simulink model "model_1_2_tasks"  (R2021b)
settings: Solver=FixedStepAuto  StartTime=0.0  StopTime=15  FixedStep=0.001  RelTol=1e-3
undefined symbols (not defined in the file): A1, A2, B1, B2, C1, C2, D1, D2, K1, K2, L1, L2
settings Model: Creator=den  LastModifiedBy=den

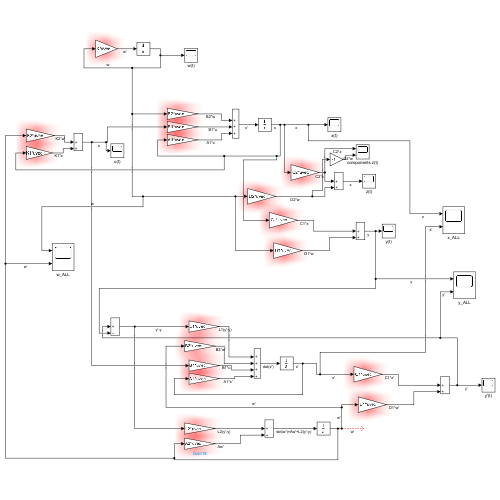
[thumbnail: Simulink's stored preview of the top-level diagram]
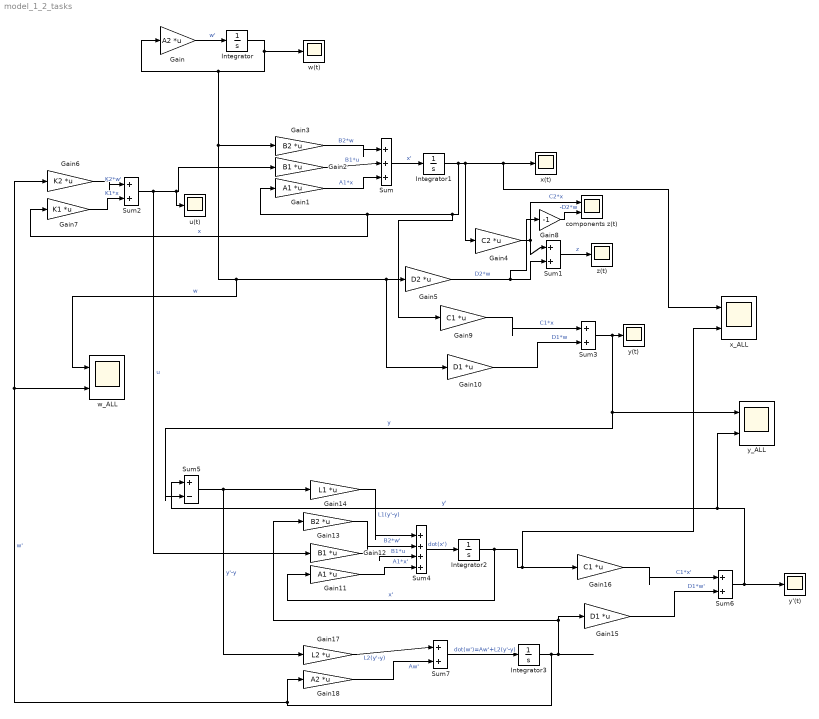
== system model_1_2_tasks ==
  Gain : Gain  Gain=A2  Multiplication=Matrix(K*u) (u vector)
  Gain1 : Gain  Gain=A1  Multiplication=Matrix(K*u) (u vector)
  Gain10 : Gain  Gain=D1  Multiplication=Matrix(K*u) (u vector)
  Gain11 : Gain  Gain=A1  Multiplication=Matrix(K*u) (u vector)
  Gain12 : Gain  Gain=B1  Multiplication=Matrix(K*u) (u vector)
  Gain13 : Gain  Gain=B2  Multiplication=Matrix(K*u) (u vector)
  Gain14 : Gain  Gain=L1  Multiplication=Matrix(K*u) (u vector)
  Gain15 : Gain  Gain=D1  Multiplication=Matrix(K*u) (u vector)
  Gain16 : Gain  Gain=C1  Multiplication=Matrix(K*u) (u vector)
  Gain17 : Gain  Gain=L2  Multiplication=Matrix(K*u) (u vector)
  Gain18 : Gain  Gain=A2  Multiplication=Matrix(K*u) (u vector)
  Gain2 : Gain  Gain=B1  Multiplication=Matrix(K*u) (u vector)
  Gain3 : Gain  Gain=B2  Multiplication=Matrix(K*u) (u vector)
  Gain4 : Gain  Gain=C2  Multiplication=Matrix(K*u) (u vector)
  Gain5 : Gain  Gain=D2  Multiplication=Matrix(K*u) (u vector)
  Gain6 : Gain  Gain=K2  Multiplication=Matrix(K*u) (u vector)
  Gain7 : Gain  Gain=K1  Multiplication=Matrix(K*u) (u vector)
  Gain8 : Gain  Gain=-1
  Gain9 : Gain  Gain=C1  Multiplication=Matrix(K*u) (u vector)
  Integrator : Integrator  InitialCondition=[1;1;1;1]
  Integrator1 : Integrator  InitialCondition=[0;0;0]
  Integrator2 : Integrator  InitialCondition=[0;0;0]
  Integrator3 : Integrator
  Sum : Sum  Inputs=|+++
  Sum{1..3,6..7} (5 alike) : Sum  Inputs=|++
  Sum4 : Sum  Inputs=|++++
  Sum5 : Sum  Inputs=|+-
  components z(t) : Scope  NumInputPorts=2
  u(t) : Scope
  w(t) : Scope
  w_ALL : Scope  NumInputPorts=2
  x(t) : Scope
  x_ALL : Scope  NumInputPorts=2
  y'(t) : Scope
  y(t) : Scope
  y_ALL : Scope  NumInputPorts=2
  z(t) : Scope
  wires:
  Gain/1 -> Integrator/1  "w'"
  Integrator/1 -> w_ALL/1, Gain10/1, Gain5/1, Gain3/1, Gain/1, w(t)/1  "w"
  Sum/1 -> Integrator1/1  "x'"
  Gain3/1 -> Sum/1  "B2*w"
  Gain1/1 -> Sum/3  "A1*x"
  Gain2/1 -> Sum/2  "B1*u"
  Integrator1/1 -> Gain4/1, x_ALL/1, x(t)/1, Gain9/1, Gain7/1, Gain1/1  "x"
  Gain4/1 -> components z(t)/1, Sum1/1  "C2*x"
  Gain5/1 -> Gain8/1, Sum1/2  "D2*w"
  Sum1/1 -> z(t)/1  "z"
  Gain7/1 -> Sum2/2  "K1*x"
  Sum2/1 -> Gain12/1, u(t)/1, Gain2/1  "u"
  Gain6/1 -> Sum2/1  "K2*w'"
  Gain8/1 -> components z(t)/2  "-D2*w"
  Gain9/1 -> Sum3/1  "C1*x"
  Gain10/1 -> Sum3/2  "D1*w"
  Sum3/1 -> y_ALL/1, Sum5/2, y(t)/1  "y"
  Gain11/1 -> Sum4/4  "A1*x'"
  Sum4/1 -> Integrator2/1  "dot(x')"
  Gain13/1 -> Sum4/2  "B2*w'"
  Gain12/1 -> Sum4/3  "B1*u"
  Integrator2/1 -> Gain11/1, x_ALL/2, Gain16/1  "x'"
  Gain14/1 -> Sum4/1  "L1(y'-y)"
  Sum5/1 -> Gain17/1, Gain14/1  "y'-y"
  Gain15/1 -> Sum6/2  "D1*w'"
  Gain16/1 -> Sum6/1  "C1*x'"
  Sum6/1 -> y_ALL/2, Sum5/1, y'(t)/1  "y'"
  Integrator3/1 -> w_ALL/2, Gain6/1, Gain18/1, Gain13/1, Gain15/1  "w'"
  Gain17/1 -> Sum7/1  "L2(y'-y)"
  Gain18/1 -> Sum7/2  "Aw'"
  Sum7/1 -> Integrator3/1  "dot(w')=Aw'+L2(y'-y)"
